simulink model "motorbrushless_simulation"  (R2013a)
settings: Solver=ode4  StartTime=0  StopTime=0.2  FixedStep=Ts  MaxStep=1e-6  RelTol=1e-6  AbsTol=1e-6
PreLoadFcn:
  | assignin('base','Ts',[5e-6])
undefined symbols (not defined in the file or in its folder): Ts
libraries: simulink x19, powerlib_meascontrol x18, powerlib x16
Description:
  | This example illustrates use of the BLDC in a closed-loop
  | speed and voltage control on a 1 kW, 3000 rpm industrial motor
  | 
  | 
  | Copyright 2008-2013 The MathWorks, Inc.
settings Model: ExtModeAutoUpdateStatusClock=off  Creator=MathWorks  LastModifiedBy=Juan Esteban
settings DataIOCC: SignalLoggingSaveFormat=ModelDataLogs  SignalLoggingName=sigsOut
settings OptimizationCC: ExpressionDepthLimit=2147483647  InitFltsAndDblsToZero=on
settings DebuggingCC: SignalResolutionControl=TryResolveAllWithWarning  SolverPrmCheckMsg=none  MultiTaskDSMMsg=warning  MultiTaskCondExecSysMsg=none  FcnCallInpInsideContextMsg=UseLocalSettings
settings HardwareCC: TargetIntDivRoundTo=Zero  TargetEndianess=LittleEndian  TargetHWDeviceType=MATLAB Host  ProdEqTarget=off
settings RTWCC: IncludeERTFirstTime=on
settings GRTTargetCC: CombineOutputUpdateFcns=off  GRTInterface=on

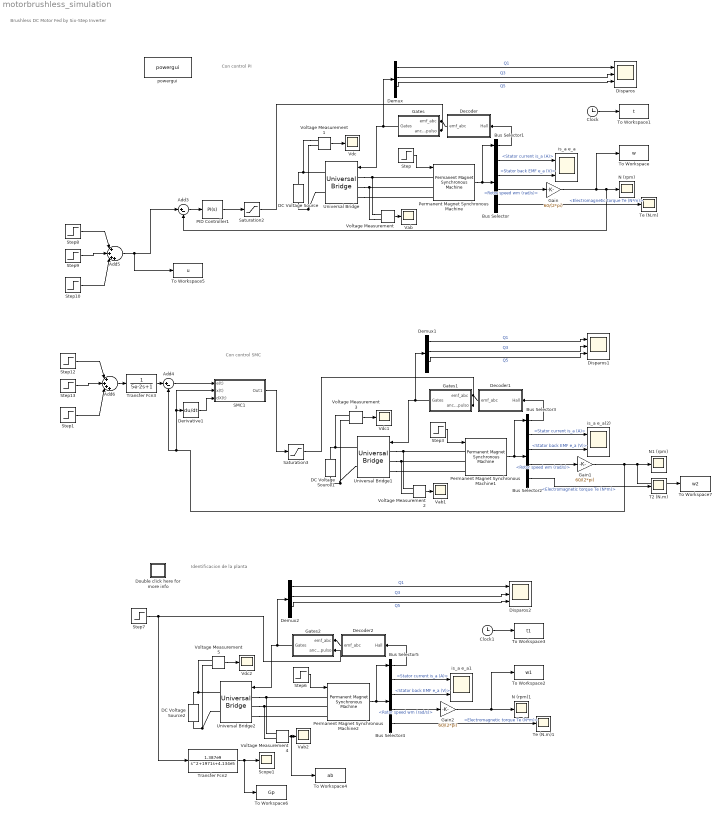
== system motorbrushless_simulation ==
  note: Identificacion de la planta
  note: Con control SMC
  note: Con control PI
  note: Brushless DC Motor Fed by Six-Step Inverter
  Add3 : Sum  Inputs=|+-
  Add4 : Sum  Inputs=|+-
  Add5 : Sum  Inputs=|++++
  Add6 : Sum  Inputs=|++++
  Bus Selector : BusSelector  OutputSignals=Stator current is_a (A),Stator back EMF e_a (V),Rotor speed wm (rad/s),Electromagnetic torque Te (N*m)
  Bus Selector1 : BusSelector  OutputSignals=Hall effect signal h_a,Hall effect signal h_b,Hall effect signal h_c  OutputAsBus=on
  Bus Selector2 : BusSelector  OutputSignals=Stator current is_a (A),Stator back EMF e_a (V),Rotor speed wm (rad/s),Electromagnetic torque Te (N*m)
  Bus Selector3 : BusSelector  OutputSignals=Hall effect signal h_a,Hall effect signal h_b,Hall effect signal h_c  OutputAsBus=on
  Bus Selector4 : BusSelector  OutputSignals=Stator current is_a (A),Stator back EMF e_a (V),Rotor speed wm (rad/s),Electromagnetic torque Te (N*m)
  Bus Selector5 : BusSelector  OutputSignals=Hall effect signal h_a,Hall effect signal h_b,Hall effect signal h_c  OutputAsBus=on
  Clock : Clock
  Clock1 : Clock
  DC Voltage Source : powerlib/Electrical Sources/DC Voltage Source  Amplitude=500  Measurements=None
  DC Voltage Source1 : powerlib/Electrical Sources/DC Voltage Source  Amplitude=500  Measurements=None
  DC Voltage Source2 : powerlib/Electrical Sources/DC Voltage Source  Amplitude=500  Measurements=None
  Decoder : Subsystem
  Decoder1 : Subsystem
  Decoder2 : Subsystem
  Demux : Demux  Outputs=6
  Demux1 : Demux  Outputs=6
  Demux2 : Demux  Outputs=6
  Derivative1 : Derivative
  Disparos : Scope  NumInputPorts=3
      settings: TimeRange=0.2  YMin=0~-5~-5  YMax=500~5~5  DataFormat=Structure
  Disparos1 : Scope  NumInputPorts=3
      settings: TimeRange=0.2  YMin=0~-5~-5  YMax=500~5~5  DataFormat=Structure
  Disparos2 : Scope  NumInputPorts=3
      settings: TimeRange=0.2  YMin=0~-5~-5  YMax=500~5~5  SaveName=ScopeData6  DataFormat=Structure
  Double click here for more info : Subsystem
      settings: OpenFcn=showdemo(bdroot(gcb))
      mask Display: disp('?')
  Gain : Gain  Gain=60/(2*pi)
  Gain1 : Gain  Gain=60/(2*pi)
  Gain2 : Gain  Gain=60/(2*pi)
  Gates : Subsystem
  Gates1 : Subsystem
  Gates2 : Subsystem
  N (rpm) : Scope
      settings: TimeRange=0.2  YMin=0  YMax=3500  SaveName=N
  N (rpm)1 : Scope
      settings: TimeRange=0.2  YMin=2000  YMax=2900  SaveName=N4
  N1 (rpm) : Scope
      settings: TimeRange=0.2  YMin=2040  YMax=2087.5  SaveName=N2
  PID Controller1 : simulink/Continuous/PID Controller  Controller=PI  TimeDomain=Continuous-time  SampleTime=1  IntegratorMethod=Forward Euler  FilterMethod=Forward Euler  Form=Ideal  P=0.000390488448665948  I=609.105574706689  D=0  N=100  InitialConditionSource=internal  InitialConditionForIntegrator=0  InitialConditionForFilter=0  ExternalReset=none  LimitOutput=off  UpperSaturationLimit=inf  LowerSaturationLimit=-inf  LinearizeAsGain=on  AntiWindupMode=none  Kb=1  TrackingMode=off  Kt=1  PParamMin=[]  PParamMax=[]  IParamMin=[]  IParamMax=[]  DParamMin=[]  DParamMax=[]  NParamMin=[]  NParamMax=[]  KbParamMin=[]  KbParamMax=[]  KtParamMin=[]  KtParamMax=[]  POutMin=[]  POutMax=[]  IOutMin=[]  IOutMax=[]  DOutMin=[]  DOutMax=[]  NOutMin=[]  NOutMax=[]  KbOutMin=[]  KbOutMax=[]  KtOutMin=[]  KtOutMax=[]  IntegratorOutMin=[]  IntegratorOutMax=[]  FilterOutMin=[]  FilterOutMax=[]  SumOutMin=[]  SumOutMax=[]  SumI1OutMin=[]  SumI1OutMax=[]  SumI2OutMin=[]  SumI2OutMax=[]  SumI3OutMin=[]  SumI3OutMax=[]  SumDOutMin=[]  SumDOutMax=[]  SaturationOutMin=[]  SaturationOutMax=[]  IntegratorContinuousStateAttributes=''  IntegratorStateMustResolveToSignalObject=off  IntegratorRTWStateStorageClass=Auto  FilterContinuousStateAttributes=''  FilterStateMustResolveToSignalObject=off  FilterRTWStateStorageClass=Auto
  Permanent Magnet Synchronous Machine : powerlib/Machines/Permanent Magnet Synchronous Machine  NbPhases=3  FluxDistribution=Trapezoidal  RotorType=Round  MechanicalLoad=Torque Tm  PresetModel=No  ShowDetailedParameters=on  Resistance=2.8750  Inductance=8.5e-3  dqInductances=[8.5e-3, 8.5e-3]  La=0.000835  MachineConstant=Flux linkage established by magnets (V.s)  Flux=0.175  VoltageCst=146.6077  TorqueCst=1.4  Flat=120  Mechanical=[ 0.8e-3, 1e-3 4]  PolePairs=4  InitialConditions=[0,0, 0,0]  InitialConditions5ph=[0 0 0 0 0 0]  TsPowergui=0  TsBlock=-1  RefAngle=90 degrees behind phase A axis (modified Park)
  Permanent Magnet Synchronous Machine1 : powerlib/Machines/Permanent Magnet Synchronous Machine  NbPhases=3  FluxDistribution=Trapezoidal  RotorType=Round  MechanicalLoad=Torque Tm  PresetModel=No  ShowDetailedParameters=on  Resistance=2.8750  Inductance=8.5e-3  dqInductances=[8.5e-3, 8.5e-3]  La=0.000835  MachineConstant=Flux linkage established by magnets (V.s)  Flux=0.175  VoltageCst=146.6077  TorqueCst=1.4  Flat=120  Mechanical=[ 0.8e-3, 1e-3 4]  PolePairs=4  InitialConditions=[0,0, 0,0]  InitialConditions5ph=[0 0 0 0 0 0]  TsPowergui=0  TsBlock=-1  RefAngle=90 degrees behind phase A axis (modified Park)
  Permanent Magnet Synchronous Machine2 : powerlib/Machines/Permanent Magnet Synchronous Machine  NbPhases=3  FluxDistribution=Trapezoidal  RotorType=Round  MechanicalLoad=Torque Tm  PresetModel=No  ShowDetailedParameters=on  Resistance=2.8750  Inductance=8.5e-3  dqInductances=[8.5e-3, 8.5e-3]  La=0.000835  MachineConstant=Flux linkage established by magnets (V.s)  Flux=0.175  VoltageCst=146.6077  TorqueCst=1.4  Flat=120  Mechanical=[ 0.8e-3, 1e-3 4]  PolePairs=4  InitialConditions=[0,0, 0,0]  InitialConditions5ph=[0 0 0 0 0 0]  TsPowergui=0  TsBlock=-1  RefAngle=90 degrees behind phase A axis (modified Park)
  SMC1 : Subsystem  TreatAsAtomicUnit=on
  Saturation2 : Saturate  UpperLimit=1  LowerLimit=0
  Saturation3 : Saturate  UpperLimit=1  LowerLimit=0
  Scope1 : Scope
      settings: SaveName=ScopeData7
  Step : Step  Time=.1  After=0  SampleTime=0
  Step1 : Step  Time=2.4  After=-2500  SampleTime=0
  Step10 : Step  Time=2.4  After=-2500  SampleTime=0
  Step12 : Step  Time=0  After=1000  SampleTime=0
  Step13 : Step  Time=1.2  After=2000  SampleTime=0
  Step3 : Step  Time=.1  After=0  SampleTime=0
  Step6 : Step  Time=.1  After=0  SampleTime=0
  Step7 : Step  Time=0  SampleTime=0
  Step8 : Step  Time=0  After=1000  SampleTime=0
  Step9 : Step  Time=1.2  After=2000  SampleTime=0
  T2 (N.m) : Scope
      settings: TimeRange=0.2  YMin=0  YMax=3500  SaveName=N3
  Te (N.m) : Scope
      settings: TimeRange=0.2  YMin=0  YMax=3500  SaveName=N1
  Te (N.m)1 : Scope
      settings: TimeRange=0.2  YMin=0  YMax=3500  SaveName=N5
  To Workspace : ToWorkspace  VariableName=w  SampleTime=-1
  To Workspace1 : ToWorkspace  VariableName=t  SampleTime=-1
  To Workspace2 : ToWorkspace  VariableName=w1  SampleTime=-1
  To Workspace3 : ToWorkspace  VariableName=t1  SampleTime=-1
  To Workspace4 : ToWorkspace  VariableName=ab  SampleTime=-1
  To Workspace5 : ToWorkspace  VariableName=u  SampleTime=-1
  To Workspace6 : ToWorkspace  VariableName=Gp  SampleTime=-1
  To Workspace7 : ToWorkspace  VariableName=w2  SampleTime=-1
  Transfer Fcn2 : TransferFcn  Numerator=[1.387e9]  Denominator=[1 1971 4.134e5]
  Transfer Fcn3 : TransferFcn  Denominator=[5e-2 1]
  Universal Bridge : powerlib/Power Electronics/Universal Bridge  Arms=3  SnubberResistance=5000  SnubberCapacitance=1e-6  Device=MOSFET / Diodes  Ron=1e-3  Lon=0  ForwardVoltages="[  0  0  ]"  ForwardVoltage=0  GTOparameters=[ 10e-6 , 20e-6 ]  IGBTparameters=[ 1e-6 , 2e-6 ]  Measurements=None  Measurements_2=None  converterType=Rectifier
  Universal Bridge1 : powerlib/Power Electronics/Universal Bridge  Arms=3  SnubberResistance=5000  SnubberCapacitance=1e-6  Device=MOSFET / Diodes  Ron=1e-3  Lon=0  ForwardVoltages="[  0  0  ]"  ForwardVoltage=0  GTOparameters=[ 10e-6 , 20e-6 ]  IGBTparameters=[ 1e-6 , 2e-6 ]  Measurements=None  Measurements_2=None  converterType=Rectifier
  Universal Bridge2 : powerlib/Power Electronics/Universal Bridge  Arms=3  SnubberResistance=5000  SnubberCapacitance=1e-6  Device=MOSFET / Diodes  Ron=1e-3  Lon=0  ForwardVoltages="[  0  0  ]"  ForwardVoltage=0  GTOparameters=[ 10e-6 , 20e-6 ]  IGBTparameters=[ 1e-6 , 2e-6 ]  Measurements=None  Measurements_2=None  converterType=Rectifier
  Vab : Scope
      settings: TimeRange=0.06  YMin=-10000  YMax=10000  SaveName=ScopeData4  DataFormat=Structure
  Vab1 : Scope
      settings: TimeRange=0.06  YMin=-10000  YMax=10000  SaveName=ScopeData2  DataFormat=Structure
  Vab2 : Scope
      settings: TimeRange=0.06  YMin=-10000  YMax=10000  SaveName=ScopeData8  DataFormat=Structure
  Vdc : Scope
      settings: TimeRange=0.2  YMin=0  YMax=500  SaveName=ScopeData3  DataFormat=Structure
  Vdc1 : Scope
      settings: TimeRange=0.2  YMin=0  YMax=500  SaveName=ScopeData5  DataFormat=Structure
  Vdc2 : Scope
      settings: TimeRange=0.2  YMin=0  YMax=500  SaveName=ScopeData9  DataFormat=Structure
  Voltage Measurement{,1..5} (6 alike) : powerlib/Measurements/Voltage Measurement  PhasorSimulation=off  OutputType=Complex  PSBequivalent=0
  is_a e_a : Scope  NumInputPorts=2
      settings: TimeRange=0.2  YMin=-15~-250  YMax=20~250  SaveName=IE
  is_a e_a(2) : Scope  NumInputPorts=2
      settings: TimeRange=0.2  YMin=-15~-250  YMax=20~250  SaveName=IE1
  is_a e_a1 : Scope  NumInputPorts=2
      settings: TimeRange=0.2  YMin=-15~-250  YMax=20~250  SaveName=IE2
  powergui : powerlib/powergui  Priority=2  SimulationMode=Discrete  SolverType=Tustin  SampleTime=Ts  frequency=60  SPID=off  DisableSnubberDevices=off  DisableRonSwitches=off  DisableVfSwitches=off  SwTol=0  Interpol=off  DisplayEquations=off  frequencyindice=0  Pbase=100e6  ErrMax=1e-4  Iterations=50  UnitsV=kV  UnitsW=MW  FunctionMessages=off  echomessages=off  HookPort=off  EnableUseOfTLC=off  x0status=blocks  RestoreLinks=warning  ResistiveCurrentMeasurement=off  Frange=[0:2:500]  Ylog=off  Xlog=on  ShowGrid=off  save=off  variable=ZData  ZoomFFT=on  StartTime=0.0  cycles=1  DisplayStyle=1  fundamental=60  FreqAxis=off  MaxFrequency=1000  frequencyindicesteady=1  RmsSteady=1  display=off  Ts=0  methode=off
  wires:
  Step/1 -> Permanent Magnet Synchronous Machine/1
  Gates/1(Gates) -> Demux/1, Universal Bridge/1
  Decoder/1(emf_abc) -> Gates/1("emf_abc ")
  Voltage Measurement/1 -> Vab/1
  Voltage Measurement1/1 -> Vdc/1
  Bus Selector/1 -> is_a e_a/1  "<Stator current is_a (A)>"
  Permanent Magnet Synchronous Machine/1 -> Bus Selector/1, Bus Selector1/1
  Bus Selector1/1 -> Decoder/1("Hall ")
  Bus Selector/2 -> is_a e_a/2  "<Stator back EMF e_a (V)>"
  Bus Selector/4 -> Te (N.m)/1  "<Electromagnetic torque Te (N*m)>"
  Bus Selector/3 -> Gain/1  "<Rotor speed wm (rad/s)>"
  Gain/1 -> To Workspace/1, Add3/2, N (rpm)/1
  Clock/1 -> To Workspace1/1
  Add3/1 -> PID Controller1/1
  Demux/1 -> Disparos/1  "Q1"
  Demux/3 -> Disparos/2  "Q3"
  Demux/5 -> Disparos/3  "Q5"
  PID Controller1/1 -> Saturation2/1
  Saturation2/1 -> Gates/2(ancho_pulso)
  Add5/1 -> To Workspace5/1, Add3/1
  Step8/1 -> Add5/1
  Step9/1 -> Add5/2
  Step10/1 -> Add5/3
  Step3/1 -> Permanent Magnet Synchronous Machine1/1
  Gates1/1(Gates) -> Demux1/1, Universal Bridge1/1
  Decoder1/1(emf_abc) -> Gates1/1("emf_abc ")
  Voltage Measurement2/1 -> Vab1/1
  Voltage Measurement3/1 -> Vdc1/1
  Bus Selector2/1 -> is_a e_a(2)/1  "<Stator current is_a (A)>"
  Permanent Magnet Synchronous Machine1/1 -> Bus Selector2/1, Bus Selector3/1
  Bus Selector3/1 -> Decoder1/1("Hall ")
  Bus Selector2/2 -> is_a e_a(2)/2  "<Stator back EMF e_a (V)>"
  Bus Selector2/4 -> T2 (N.m)/1  "<Electromagnetic torque Te (N*m)>"
  Bus Selector2/3 -> Gain1/1  "<Rotor speed wm (rad/s)>"
  Demux1/1 -> Disparos1/1  "Q1"
  Demux1/3 -> Disparos1/2  "Q3"
  Demux1/5 -> Disparos1/3  "Q5"
  Add4/1 -> SMC1/1(e(t))
  Derivative1/1 -> SMC1/3(dX(t))
  Gain1/1 -> Derivative1/1, SMC1/2(x(t)), Add4/2, To Workspace7/1, N1 (rpm)/1
  SMC1/1(Out1) -> Saturation3/1
  Saturation3/1 -> Gates1/2(ancho_pulso)
  Step12/1 -> Add6/1
  Step13/1 -> Add6/2
  Step1/1 -> Add6/3
  Transfer Fcn3/1 -> Add4/1
  Add6/1 -> Transfer Fcn3/1
  Step6/1 -> Permanent Magnet Synchronous Machine2/1
  Gates2/1(Gates) -> Demux2/1, Universal Bridge2/1
  Decoder2/1(emf_abc) -> Gates2/1("emf_abc ")
  Voltage Measurement4/1 -> To Workspace4/1, Vab2/1
  Voltage Measurement5/1 -> Vdc2/1
  Bus Selector4/1 -> is_a e_a1/1  "<Stator current is_a (A)>"
  Permanent Magnet Synchronous Machine2/1 -> Bus Selector4/1, Bus Selector5/1
  Bus Selector5/1 -> Decoder2/1("Hall ")
  Bus Selector4/2 -> is_a e_a1/2  "<Stator back EMF e_a (V)>"
  Bus Selector4/4 -> Te (N.m)1/1  "<Electromagnetic torque Te (N*m)>"
  Bus Selector4/3 -> Gain2/1  "<Rotor speed wm (rad/s)>"
  Gain2/1 -> To Workspace2/1, N (rpm)1/1
  Clock1/1 -> To Workspace3/1
  Demux2/1 -> Disparos2/1  "Q1"
  Demux2/3 -> Disparos2/2  "Q3"
  Demux2/5 -> Disparos2/3  "Q5"
  Step7/1 -> Transfer Fcn2/1, Gates2/2(ancho_pulso)
  Transfer Fcn2/1 -> To Workspace6/1, Scope1/1
  connections:
  Voltage Measurement/LConn1 -- Permanent Magnet Synchronous Machine/LConn1 -- Universal Bridge/LConn1
  Voltage Measurement/LConn2 -- Permanent Magnet Synchronous Machine/LConn2 -- Universal Bridge/LConn2
  Voltage Measurement1/LConn1 -- Universal Bridge/RConn1 -- DC Voltage Source/RConn1
  Voltage Measurement1/LConn2 -- Universal Bridge/RConn2 -- DC Voltage Source/LConn1
  Universal Bridge/LConn3 -- Permanent Magnet Synchronous Machine/LConn3
  Universal Bridge1/LConn1 -- Voltage Measurement2/LConn1 -- Permanent Magnet Synchronous Machine1/LConn1
  Universal Bridge1/LConn2 -- Voltage Measurement2/LConn2 -- Permanent Magnet Synchronous Machine1/LConn2
  DC Voltage Source1/RConn1 -- Voltage Measurement3/LConn1 -- Universal Bridge1/RConn1
  DC Voltage Source1/LConn1 -- Voltage Measurement3/LConn2 -- Universal Bridge1/RConn2
  Universal Bridge1/LConn3 -- Permanent Magnet Synchronous Machine1/LConn3
  Universal Bridge2/LConn1 -- Voltage Measurement4/LConn1 -- Permanent Magnet Synchronous Machine2/LConn1
  Universal Bridge2/LConn2 -- Voltage Measurement4/LConn2 -- Permanent Magnet Synchronous Machine2/LConn2
  DC Voltage Source2/RConn1 -- Voltage Measurement5/LConn1 -- Universal Bridge2/RConn1
  DC Voltage Source2/LConn1 -- Voltage Measurement5/LConn2 -- Universal Bridge2/RConn2
  Universal Bridge2/LConn3 -- Permanent Magnet Synchronous Machine2/LConn3

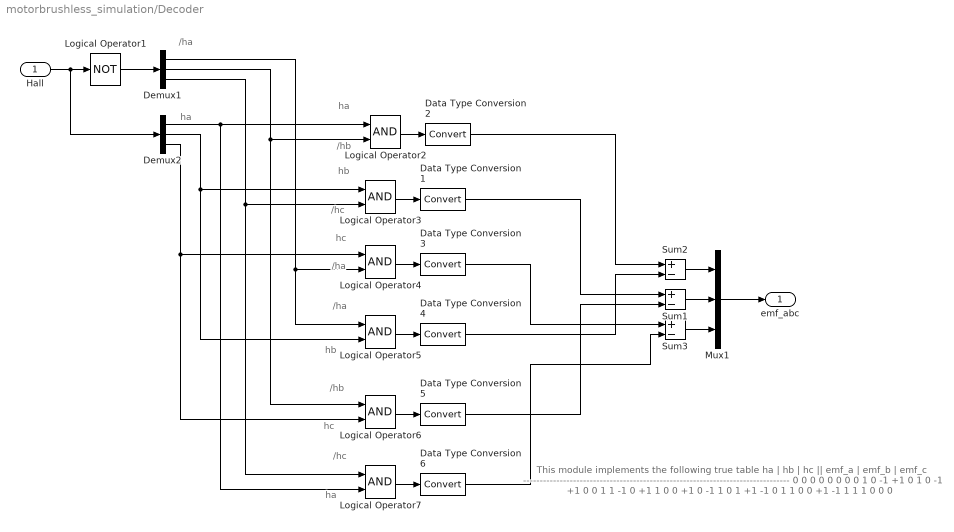
== system motorbrushless_simulation/Decoder ==
  note: /ha
  note: ha
  note: ha
  note: /hb
  note: hb
  note: /hc
  note: hc
  note: /ha
  note: /ha
  note: hb
  note: /hb
  note: hc
  note: /hc
  note: ha
  note: This module implements the following true table
      |
      |    ha   |   hb   |   hc   ||   emf_a   |   emf_b   |   emf_c
      |     --------------------------------------------------------------------------------
      | 0          0         0          0               0               0
      | 0          0         1          0               -1              +1
      | 0          1         0          -1              +1                0
      | 0          1         1          -1               0               +1
      | 1          0         0         +1               0               -1
      | 1          0         1         +1              -1                0
      | 1          1         0          0              +1               -1
      | 1          1         1          0               0                0
  "Hall " : Inport
  Data Type Conversion{1..6} (6 alike) : DataTypeConversion
  Demux1 : Demux  Outputs=3
  Demux2 : Demux  Outputs=3
  Logical Operator1 : Logic  Operator=NOT  AllPortsSameDT=off  OutDataTypeStr=boolean
  Logical Operator{2..7} (6 alike) : Logic  AllPortsSameDT=off  OutDataTypeStr=boolean
  Mux1 : Mux  Inputs=3
  Sum1 : Sum  Inputs=+-  OutDataTypeStr=double
  Sum2 : Sum  Inputs=+-  OutDataTypeStr=double
  Sum3 : Sum  Inputs=+-  OutDataTypeStr=double
  emf_abc : Outport
  wires:
  "Hall "/1 -> Logical Operator1/1, Demux2/1
  Logical Operator1/1 -> Demux1/1
  Demux2/3 -> Logical Operator4/1, Logical Operator6/2
  Demux2/2 -> Logical Operator3/1, Logical Operator5/2
  Demux2/1 -> Logical Operator2/1, Logical Operator7/2
  Demux1/3 -> Logical Operator3/2, Logical Operator7/1
  Demux1/2 -> Logical Operator2/2, Logical Operator6/1
  Demux1/1 -> Logical Operator4/2, Logical Operator5/1
  Logical Operator2/1 -> Data Type Conversion2/1
  Sum2/1 -> Mux1/1
  Sum1/1 -> Mux1/2
  Sum3/1 -> Mux1/3
  Mux1/1 -> emf_abc/1
  Logical Operator3/1 -> Data Type Conversion1/1
  Logical Operator4/1 -> Data Type Conversion3/1
  Logical Operator5/1 -> Data Type Conversion4/1
  Logical Operator6/1 -> Data Type Conversion5/1
  Logical Operator7/1 -> Data Type Conversion6/1
  Data Type Conversion2/1 -> Sum2/1
  Data Type Conversion4/1 -> Sum2/2
  Data Type Conversion1/1 -> Sum1/1
  Data Type Conversion5/1 -> Sum1/2
  Data Type Conversion3/1 -> Sum3/1
  Data Type Conversion6/1 -> Sum3/2

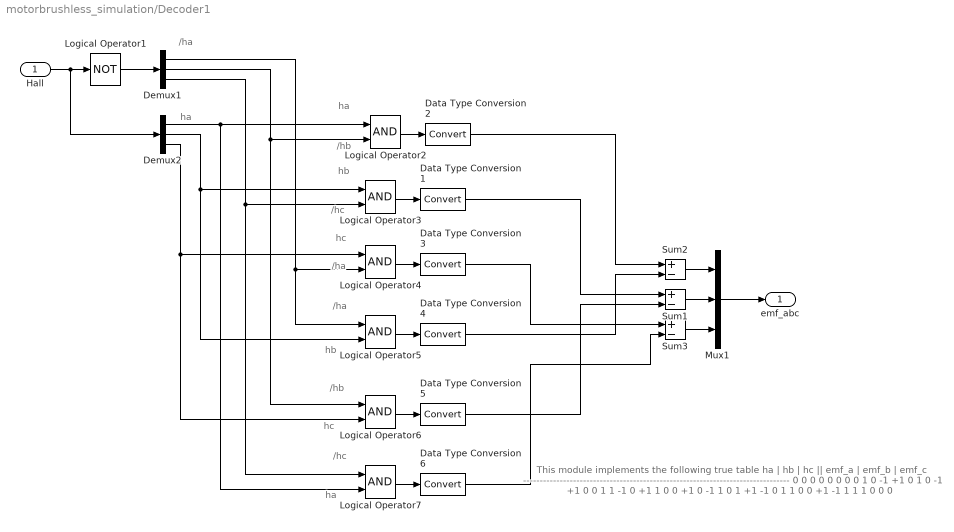
== system motorbrushless_simulation/Decoder1 ==
  note: /ha
  note: ha
  note: ha
  note: /hb
  note: hb
  note: /hc
  note: hc
  note: /ha
  note: /ha
  note: hb
  note: /hb
  note: hc
  note: /hc
  note: ha
  note: This module implements the following true table
      |
      |    ha   |   hb   |   hc   ||   emf_a   |   emf_b   |   emf_c
      |     --------------------------------------------------------------------------------
      | 0          0         0          0               0               0
      | 0          0         1          0               -1              +1
      | 0          1         0          -1              +1                0
      | 0          1         1          -1               0               +1
      | 1          0         0         +1               0               -1
      | 1          0         1         +1              -1                0
      | 1          1         0          0              +1               -1
      | 1          1         1          0               0                0
  "Hall " : Inport
  Data Type Conversion{1..6} (6 alike) : DataTypeConversion
  Demux1 : Demux  Outputs=3
  Demux2 : Demux  Outputs=3
  Logical Operator1 : Logic  Operator=NOT  AllPortsSameDT=off  OutDataTypeStr=boolean
  Logical Operator{2..7} (6 alike) : Logic  AllPortsSameDT=off  OutDataTypeStr=boolean
  Mux1 : Mux  Inputs=3
  Sum1 : Sum  Inputs=+-  OutDataTypeStr=double
  Sum2 : Sum  Inputs=+-  OutDataTypeStr=double
  Sum3 : Sum  Inputs=+-  OutDataTypeStr=double
  emf_abc : Outport
  wires:
  "Hall "/1 -> Logical Operator1/1, Demux2/1
  Logical Operator1/1 -> Demux1/1
  Demux2/3 -> Logical Operator4/1, Logical Operator6/2
  Demux2/2 -> Logical Operator3/1, Logical Operator5/2
  Demux2/1 -> Logical Operator2/1, Logical Operator7/2
  Demux1/3 -> Logical Operator3/2, Logical Operator7/1
  Demux1/2 -> Logical Operator2/2, Logical Operator6/1
  Demux1/1 -> Logical Operator4/2, Logical Operator5/1
  Logical Operator2/1 -> Data Type Conversion2/1
  Sum2/1 -> Mux1/1
  Sum1/1 -> Mux1/2
  Sum3/1 -> Mux1/3
  Mux1/1 -> emf_abc/1
  Logical Operator3/1 -> Data Type Conversion1/1
  Logical Operator4/1 -> Data Type Conversion3/1
  Logical Operator5/1 -> Data Type Conversion4/1
  Logical Operator6/1 -> Data Type Conversion5/1
  Logical Operator7/1 -> Data Type Conversion6/1
  Data Type Conversion2/1 -> Sum2/1
  Data Type Conversion4/1 -> Sum2/2
  Data Type Conversion1/1 -> Sum1/1
  Data Type Conversion5/1 -> Sum1/2
  Data Type Conversion3/1 -> Sum3/1
  Data Type Conversion6/1 -> Sum3/2

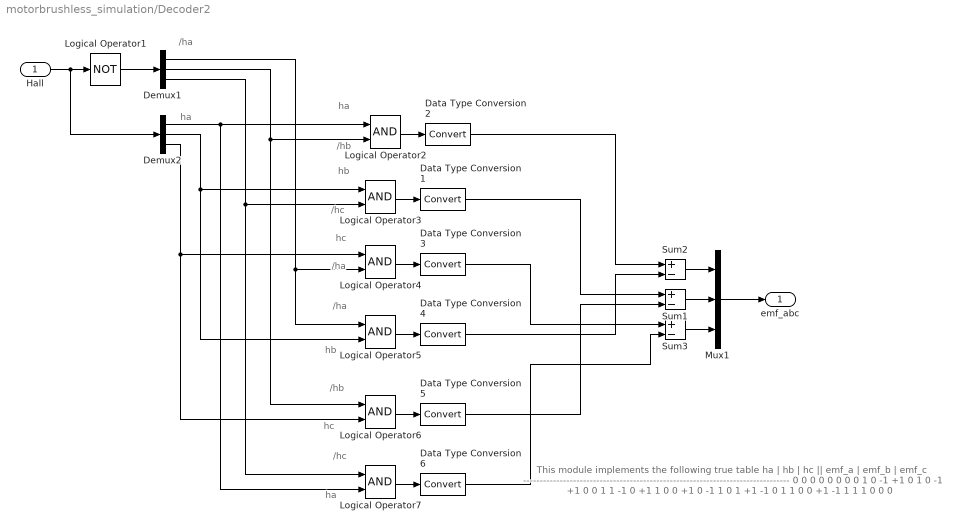
== system motorbrushless_simulation/Decoder2 ==
  note: /ha
  note: ha
  note: ha
  note: /hb
  note: hb
  note: /hc
  note: hc
  note: /ha
  note: /ha
  note: hb
  note: /hb
  note: hc
  note: /hc
  note: ha
  note: This module implements the following true table
      |
      |    ha   |   hb   |   hc   ||   emf_a   |   emf_b   |   emf_c
      |     --------------------------------------------------------------------------------
      | 0          0         0          0               0               0
      | 0          0         1          0               -1              +1
      | 0          1         0          -1              +1                0
      | 0          1         1          -1               0               +1
      | 1          0         0         +1               0               -1
      | 1          0         1         +1              -1                0
      | 1          1         0          0              +1               -1
      | 1          1         1          0               0                0
  "Hall " : Inport
  Data Type Conversion{1..6} (6 alike) : DataTypeConversion
  Demux1 : Demux  Outputs=3
  Demux2 : Demux  Outputs=3
  Logical Operator1 : Logic  Operator=NOT  AllPortsSameDT=off  OutDataTypeStr=boolean
  Logical Operator{2..7} (6 alike) : Logic  AllPortsSameDT=off  OutDataTypeStr=boolean
  Mux1 : Mux  Inputs=3
  Sum1 : Sum  Inputs=+-  OutDataTypeStr=double
  Sum2 : Sum  Inputs=+-  OutDataTypeStr=double
  Sum3 : Sum  Inputs=+-  OutDataTypeStr=double
  emf_abc : Outport
  wires:
  "Hall "/1 -> Logical Operator1/1, Demux2/1
  Logical Operator1/1 -> Demux1/1
  Demux2/3 -> Logical Operator4/1, Logical Operator6/2
  Demux2/2 -> Logical Operator3/1, Logical Operator5/2
  Demux2/1 -> Logical Operator2/1, Logical Operator7/2
  Demux1/3 -> Logical Operator3/2, Logical Operator7/1
  Demux1/2 -> Logical Operator2/2, Logical Operator6/1
  Demux1/1 -> Logical Operator4/2, Logical Operator5/1
  Logical Operator2/1 -> Data Type Conversion2/1
  Sum2/1 -> Mux1/1
  Sum1/1 -> Mux1/2
  Sum3/1 -> Mux1/3
  Mux1/1 -> emf_abc/1
  Logical Operator3/1 -> Data Type Conversion1/1
  Logical Operator4/1 -> Data Type Conversion3/1
  Logical Operator5/1 -> Data Type Conversion4/1
  Logical Operator6/1 -> Data Type Conversion5/1
  Logical Operator7/1 -> Data Type Conversion6/1
  Data Type Conversion2/1 -> Sum2/1
  Data Type Conversion4/1 -> Sum2/2
  Data Type Conversion1/1 -> Sum1/1
  Data Type Conversion5/1 -> Sum1/2
  Data Type Conversion3/1 -> Sum3/1
  Data Type Conversion6/1 -> Sum3/2

== system motorbrushless_simulation/Double click here for more info ==

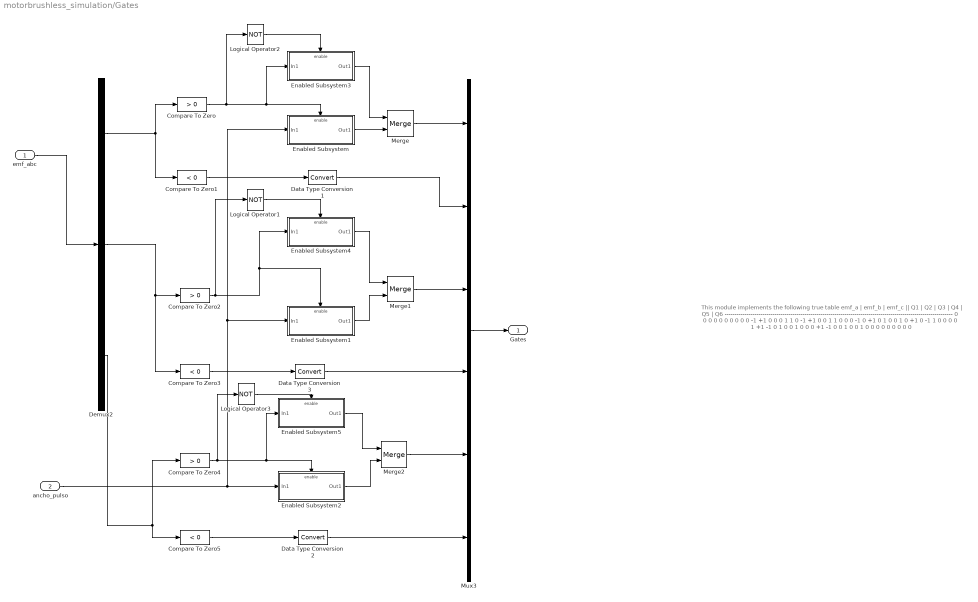
== system motorbrushless_simulation/Gates ==
  note: This module implements the following true table
      |
      |    emf_a   |   emf_b   |   emf_c   ||   Q1   |   Q2   |   Q3   |   Q4   |   Q5   |   Q6
      |     ------------------------------------------------------------------------------------------------------------------
      |       0              0                0            0          0          0           0        0        0
      |       0               -1              +1          0          0          0           1        1        0
      |     -1              +1                0          0          1          1           0        0        0
      |     -1               0               +1          0          1         0           0        1        0
      |    +1               0                -1          1          0          0           0        0        1
      |    +1              -1                0           1          0          0           1        0        0
      |      0              +1               -1           0          0          1           0        0        1
      |     0              0                0             0          0          0           0        0        0
  "emf_abc " : Inport
  ancho_pulso : Inport  Port=2
  Compare To Zero : simulink/Logic and Bit Operations/Compare To Zero  relop=>  OutDataTypeStr=boolean  ZeroCross=off
  Compare To Zero1 : simulink/Logic and Bit Operations/Compare To Zero  relop=<  OutDataTypeStr=boolean  ZeroCross=off
  Compare To Zero2 : simulink/Logic and Bit Operations/Compare To Zero  relop=>  OutDataTypeStr=boolean  ZeroCross=off
  Compare To Zero3 : simulink/Logic and Bit Operations/Compare To Zero  relop=<  OutDataTypeStr=boolean  ZeroCross=off
  Compare To Zero4 : simulink/Logic and Bit Operations/Compare To Zero  relop=>  OutDataTypeStr=boolean  ZeroCross=off
  Compare To Zero5 : simulink/Logic and Bit Operations/Compare To Zero  relop=<  OutDataTypeStr=boolean  ZeroCross=off
  Data Type Conversion1 : DataTypeConversion
  Data Type Conversion2 : DataTypeConversion
  Data Type Conversion3 : DataTypeConversion
  Demux2 : Demux  Outputs=3
  Enabled Subsystem : Subsystem  TreatAsAtomicUnit=on
  Enabled Subsystem1 : Subsystem  TreatAsAtomicUnit=on
  Enabled Subsystem2 : Subsystem  TreatAsAtomicUnit=on
  Enabled Subsystem3 : Subsystem  TreatAsAtomicUnit=on
  Enabled Subsystem4 : Subsystem  TreatAsAtomicUnit=on
  Enabled Subsystem5 : Subsystem  TreatAsAtomicUnit=on
  Logical Operator1 : Logic  Operator=NOT  Inputs=3  AllPortsSameDT=off  OutDataTypeStr=boolean
  Logical Operator2 : Logic  Operator=NOT  Inputs=3  AllPortsSameDT=off  OutDataTypeStr=boolean
  Logical Operator3 : Logic  Operator=NOT  Inputs=3  AllPortsSameDT=off  OutDataTypeStr=boolean
  Merge : Merge
  Merge1 : Merge
  Merge2 : Merge
  Mux3 : Mux  Inputs=6
  Gates : Outport
  wires:
  "emf_abc "/1 -> Demux2/1
  Mux3/1 -> Gates/1
  Demux2/1 -> Compare To Zero/1, Compare To Zero1/1
  Demux2/2 -> Compare To Zero2/1, Compare To Zero3/1
  Demux2/3 -> Compare To Zero4/1, Compare To Zero5/1
  Compare To Zero/1 -> Logical Operator2/1, Enabled Subsystem3/1(In1), Enabled Subsystem/Enable
  Enabled Subsystem/1(Out1) -> Merge/2
  Merge/1 -> Mux3/1
  Enabled Subsystem1/1(Out1) -> Merge1/2
  Merge1/1 -> Mux3/3
  Enabled Subsystem2/1(Out1) -> Merge2/2
  Merge2/1 -> Mux3/5
  Logical Operator2/1 -> Enabled Subsystem3/Enable
  Enabled Subsystem3/1(Out1) -> Merge/1
  Compare To Zero1/1 -> Data Type Conversion1/1
  Data Type Conversion1/1 -> Mux3/2
  Compare To Zero2/1 -> Enabled Subsystem4/1(In1), Enabled Subsystem1/Enable, Logical Operator1/1
  Logical Operator1/1 -> Enabled Subsystem4/Enable
  Enabled Subsystem4/1(Out1) -> Merge1/1
  Data Type Conversion3/1 -> Mux3/4
  Compare To Zero3/1 -> Data Type Conversion3/1
  Compare To Zero4/1 -> Logical Operator3/1, Enabled Subsystem5/1(In1), Enabled Subsystem2/Enable
  Logical Operator3/1 -> Enabled Subsystem5/Enable
  Compare To Zero5/1 -> Data Type Conversion2/1
  Data Type Conversion2/1 -> Mux3/6
  ancho_pulso/1 -> Enabled Subsystem1/1(In1), Enabled Subsystem/1(In1), Enabled Subsystem2/1(In1)
  Enabled Subsystem5/1(Out1) -> Merge2/1

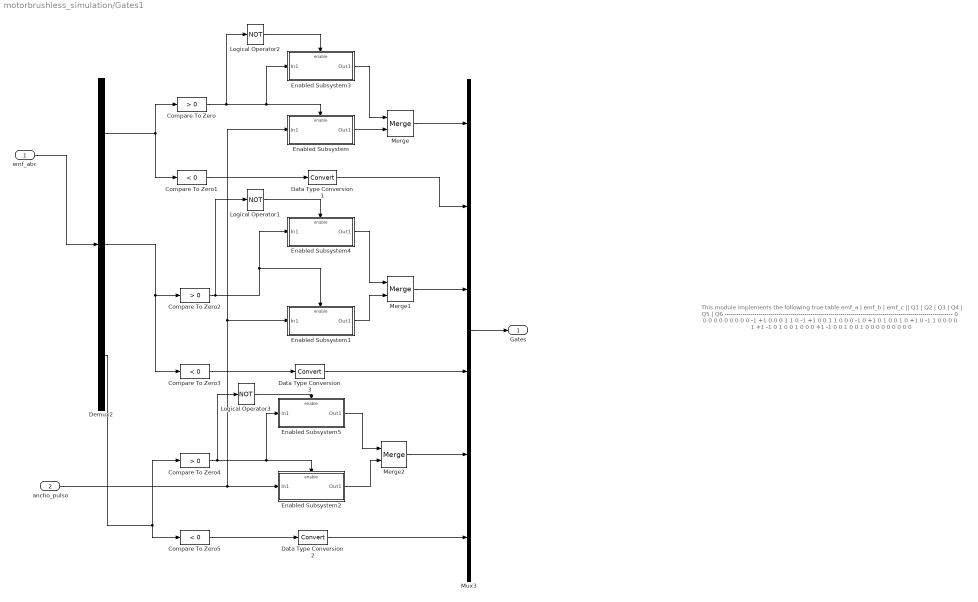
== system motorbrushless_simulation/Gates1 ==
  note: This module implements the following true table
      |
      |    emf_a   |   emf_b   |   emf_c   ||   Q1   |   Q2   |   Q3   |   Q4   |   Q5   |   Q6
      |     ------------------------------------------------------------------------------------------------------------------
      |       0              0                0            0          0          0           0        0        0
      |       0               -1              +1          0          0          0           1        1        0
      |     -1              +1                0          0          1          1           0        0        0
      |     -1               0               +1          0          1         0           0        1        0
      |    +1               0                -1          1          0          0           0        0        1
      |    +1              -1                0           1          0          0           1        0        0
      |      0              +1               -1           0          0          1           0        0        1
      |     0              0                0             0          0          0           0        0        0
  "emf_abc " : Inport
  ancho_pulso : Inport  Port=2
  Compare To Zero : simulink/Logic and Bit Operations/Compare To Zero  relop=>  OutDataTypeStr=boolean  ZeroCross=off
  Compare To Zero1 : simulink/Logic and Bit Operations/Compare To Zero  relop=<  OutDataTypeStr=boolean  ZeroCross=off
  Compare To Zero2 : simulink/Logic and Bit Operations/Compare To Zero  relop=>  OutDataTypeStr=boolean  ZeroCross=off
  Compare To Zero3 : simulink/Logic and Bit Operations/Compare To Zero  relop=<  OutDataTypeStr=boolean  ZeroCross=off
  Compare To Zero4 : simulink/Logic and Bit Operations/Compare To Zero  relop=>  OutDataTypeStr=boolean  ZeroCross=off
  Compare To Zero5 : simulink/Logic and Bit Operations/Compare To Zero  relop=<  OutDataTypeStr=boolean  ZeroCross=off
  Data Type Conversion1 : DataTypeConversion
  Data Type Conversion2 : DataTypeConversion
  Data Type Conversion3 : DataTypeConversion
  Demux2 : Demux  Outputs=3
  Enabled Subsystem : Subsystem  TreatAsAtomicUnit=on
  Enabled Subsystem1 : Subsystem  TreatAsAtomicUnit=on
  Enabled Subsystem2 : Subsystem  TreatAsAtomicUnit=on
  Enabled Subsystem3 : Subsystem  TreatAsAtomicUnit=on
  Enabled Subsystem4 : Subsystem  TreatAsAtomicUnit=on
  Enabled Subsystem5 : Subsystem  TreatAsAtomicUnit=on
  Logical Operator1 : Logic  Operator=NOT  Inputs=3  AllPortsSameDT=off  OutDataTypeStr=boolean
  Logical Operator2 : Logic  Operator=NOT  Inputs=3  AllPortsSameDT=off  OutDataTypeStr=boolean
  Logical Operator3 : Logic  Operator=NOT  Inputs=3  AllPortsSameDT=off  OutDataTypeStr=boolean
  Merge : Merge
  Merge1 : Merge
  Merge2 : Merge
  Mux3 : Mux  Inputs=6
  Gates : Outport
  wires:
  "emf_abc "/1 -> Demux2/1
  Mux3/1 -> Gates/1
  Demux2/1 -> Compare To Zero/1, Compare To Zero1/1
  Demux2/2 -> Compare To Zero2/1, Compare To Zero3/1
  Demux2/3 -> Compare To Zero4/1, Compare To Zero5/1
  Compare To Zero/1 -> Logical Operator2/1, Enabled Subsystem3/1(In1), Enabled Subsystem/Enable
  Enabled Subsystem/1(Out1) -> Merge/2
  Merge/1 -> Mux3/1
  Enabled Subsystem1/1(Out1) -> Merge1/2
  Merge1/1 -> Mux3/3
  Enabled Subsystem2/1(Out1) -> Merge2/2
  Merge2/1 -> Mux3/5
  Logical Operator2/1 -> Enabled Subsystem3/Enable
  Enabled Subsystem3/1(Out1) -> Merge/1
  Compare To Zero1/1 -> Data Type Conversion1/1
  Data Type Conversion1/1 -> Mux3/2
  Compare To Zero2/1 -> Enabled Subsystem4/1(In1), Enabled Subsystem1/Enable, Logical Operator1/1
  Logical Operator1/1 -> Enabled Subsystem4/Enable
  Enabled Subsystem4/1(Out1) -> Merge1/1
  Data Type Conversion3/1 -> Mux3/4
  Compare To Zero3/1 -> Data Type Conversion3/1
  Compare To Zero4/1 -> Logical Operator3/1, Enabled Subsystem5/1(In1), Enabled Subsystem2/Enable
  Logical Operator3/1 -> Enabled Subsystem5/Enable
  Compare To Zero5/1 -> Data Type Conversion2/1
  Data Type Conversion2/1 -> Mux3/6
  ancho_pulso/1 -> Enabled Subsystem1/1(In1), Enabled Subsystem/1(In1), Enabled Subsystem2/1(In1)
  Enabled Subsystem5/1(Out1) -> Merge2/1

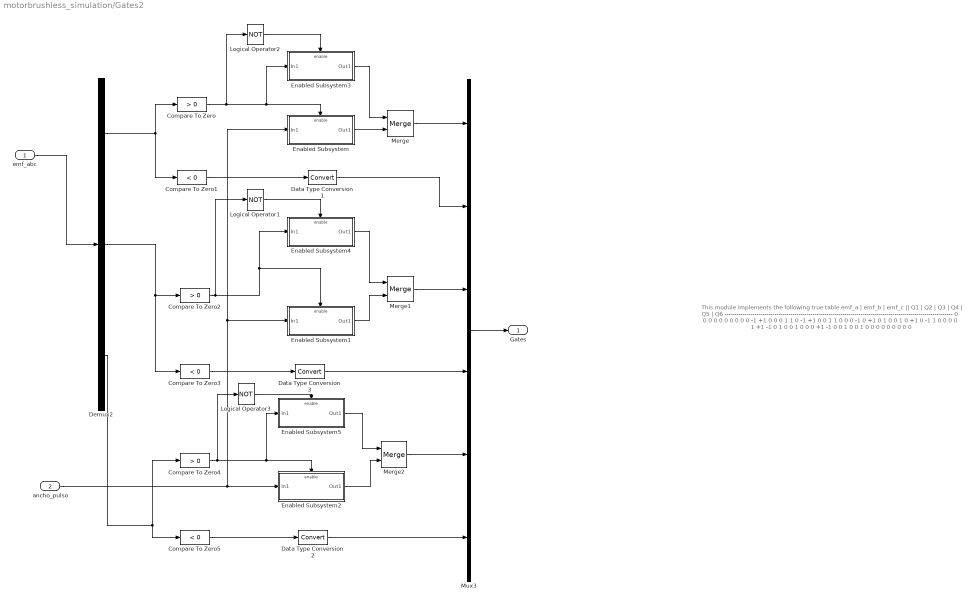
== system motorbrushless_simulation/Gates2 ==
  note: This module implements the following true table
      |
      |    emf_a   |   emf_b   |   emf_c   ||   Q1   |   Q2   |   Q3   |   Q4   |   Q5   |   Q6
      |     ------------------------------------------------------------------------------------------------------------------
      |       0              0                0            0          0          0           0        0        0
      |       0               -1              +1          0          0          0           1        1        0
      |     -1              +1                0          0          1          1           0        0        0
      |     -1               0               +1          0          1         0           0        1        0
      |    +1               0                -1          1          0          0           0        0        1
      |    +1              -1                0           1          0          0           1        0        0
      |      0              +1               -1           0          0          1           0        0        1
      |     0              0                0             0          0          0           0        0        0
  "emf_abc " : Inport
  ancho_pulso : Inport  Port=2
  Compare To Zero : simulink/Logic and Bit Operations/Compare To Zero  relop=>  OutDataTypeStr=boolean  ZeroCross=off
  Compare To Zero1 : simulink/Logic and Bit Operations/Compare To Zero  relop=<  OutDataTypeStr=boolean  ZeroCross=off
  Compare To Zero2 : simulink/Logic and Bit Operations/Compare To Zero  relop=>  OutDataTypeStr=boolean  ZeroCross=off
  Compare To Zero3 : simulink/Logic and Bit Operations/Compare To Zero  relop=<  OutDataTypeStr=boolean  ZeroCross=off
  Compare To Zero4 : simulink/Logic and Bit Operations/Compare To Zero  relop=>  OutDataTypeStr=boolean  ZeroCross=off
  Compare To Zero5 : simulink/Logic and Bit Operations/Compare To Zero  relop=<  OutDataTypeStr=boolean  ZeroCross=off
  Data Type Conversion1 : DataTypeConversion
  Data Type Conversion2 : DataTypeConversion
  Data Type Conversion3 : DataTypeConversion
  Demux2 : Demux  Outputs=3
  Enabled Subsystem : Subsystem  TreatAsAtomicUnit=on
  Enabled Subsystem1 : Subsystem  TreatAsAtomicUnit=on
  Enabled Subsystem2 : Subsystem  TreatAsAtomicUnit=on
  Enabled Subsystem3 : Subsystem  TreatAsAtomicUnit=on
  Enabled Subsystem4 : Subsystem  TreatAsAtomicUnit=on
  Enabled Subsystem5 : Subsystem  TreatAsAtomicUnit=on
  Logical Operator1 : Logic  Operator=NOT  Inputs=3  AllPortsSameDT=off  OutDataTypeStr=boolean
  Logical Operator2 : Logic  Operator=NOT  Inputs=3  AllPortsSameDT=off  OutDataTypeStr=boolean
  Logical Operator3 : Logic  Operator=NOT  Inputs=3  AllPortsSameDT=off  OutDataTypeStr=boolean
  Merge : Merge
  Merge1 : Merge
  Merge2 : Merge
  Mux3 : Mux  Inputs=6
  Gates : Outport
  wires:
  "emf_abc "/1 -> Demux2/1
  Mux3/1 -> Gates/1
  Demux2/1 -> Compare To Zero/1, Compare To Zero1/1
  Demux2/2 -> Compare To Zero2/1, Compare To Zero3/1
  Demux2/3 -> Compare To Zero4/1, Compare To Zero5/1
  Compare To Zero/1 -> Logical Operator2/1, Enabled Subsystem3/1(In1), Enabled Subsystem/Enable
  Enabled Subsystem/1(Out1) -> Merge/2
  Merge/1 -> Mux3/1
  Enabled Subsystem1/1(Out1) -> Merge1/2
  Merge1/1 -> Mux3/3
  Enabled Subsystem2/1(Out1) -> Merge2/2
  Merge2/1 -> Mux3/5
  Logical Operator2/1 -> Enabled Subsystem3/Enable
  Enabled Subsystem3/1(Out1) -> Merge/1
  Compare To Zero1/1 -> Data Type Conversion1/1
  Data Type Conversion1/1 -> Mux3/2
  Compare To Zero2/1 -> Enabled Subsystem4/1(In1), Enabled Subsystem1/Enable, Logical Operator1/1
  Logical Operator1/1 -> Enabled Subsystem4/Enable
  Enabled Subsystem4/1(Out1) -> Merge1/1
  Data Type Conversion3/1 -> Mux3/4
  Compare To Zero3/1 -> Data Type Conversion3/1
  Compare To Zero4/1 -> Logical Operator3/1, Enabled Subsystem5/1(In1), Enabled Subsystem2/Enable
  Logical Operator3/1 -> Enabled Subsystem5/Enable
  Compare To Zero5/1 -> Data Type Conversion2/1
  Data Type Conversion2/1 -> Mux3/6
  ancho_pulso/1 -> Enabled Subsystem1/1(In1), Enabled Subsystem/1(In1), Enabled Subsystem2/1(In1)
  Enabled Subsystem5/1(Out1) -> Merge2/1

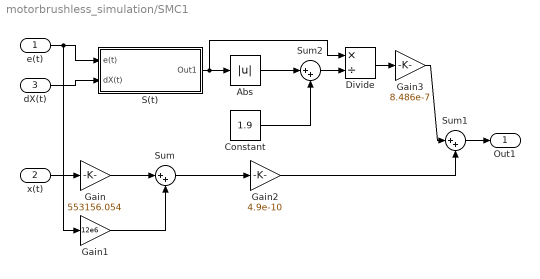
== system motorbrushless_simulation/SMC1 ==
  e(t) : Inport
  x(t) : Inport  Port=2
  dX(t) : Inport  Port=3
  Abs : Abs
  Constant : Constant  Value=1.9
  Divide : Product  Inputs=*/
  Gain : Gain  Gain=553156.054
  Gain1 : Gain  Gain=12e6
  Gain2 : Gain  Gain=4.9e-10
  Gain3 : Gain  Gain=8.486e-7
  S(t) : Subsystem  TreatAsAtomicUnit=on
  Sum : Sum  Inputs=|++
  Sum1 : Sum  Inputs=|++
  Sum2 : Sum  Inputs=|++
  Out1 : Outport
  wires:
  e(t)/1 -> Gain1/1, S(t)/1(e(t))
  dX(t)/1 -> S(t)/2(dX(t))
  x(t)/1 -> Gain/1
  Gain/1 -> Sum/1
  Gain1/1 -> Sum/2
  S(t)/1(Out1) -> Divide/1, Abs/1
  Abs/1 -> Sum2/1
  Constant/1 -> Sum2/2
  Sum2/1 -> Divide/2
  Divide/1 -> Gain3/1
  Gain3/1 -> Sum1/1
  Sum1/1 -> Out1/1
  Sum/1 -> Gain2/1
  Gain2/1 -> Sum1/2

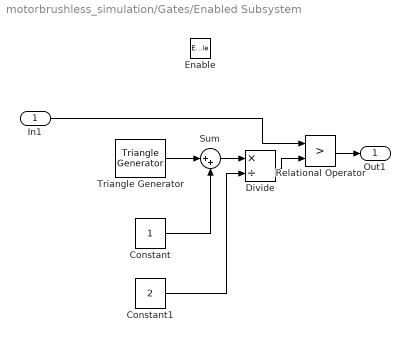
== system motorbrushless_simulation/Gates/Enabled Subsystem ==
  In1 : Inport
  Enable : EnablePort
  Constant : Constant
  Constant1 : Constant  Value=2
  Divide : Product  Inputs=*/
  Relational Operator : RelationalOperator  Operator=>  OutDataTypeStr=boolean
  Sum : Sum  Inputs=|++
  Triangle Generator : powerlib_meascontrol/Pulse & Signal Generators/Triangle Generator  Freq=4e3  Phase=90  Ts=Ts
  Out1 : Outport
  wires:
  Triangle Generator/1 -> Sum/1
  Constant/1 -> Sum/2
  Sum/1 -> Divide/1
  Divide/1 -> Relational Operator/2
  Constant1/1 -> Divide/2
  In1/1 -> Relational Operator/1
  Relational Operator/1 -> Out1/1

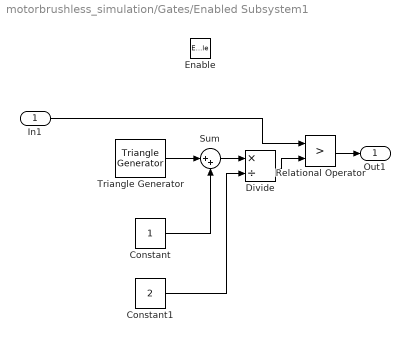
== system motorbrushless_simulation/Gates/Enabled Subsystem1 ==
  In1 : Inport
  Enable : EnablePort
  Constant : Constant
  Constant1 : Constant  Value=2
  Divide : Product  Inputs=*/
  Relational Operator : RelationalOperator  Operator=>  OutDataTypeStr=boolean
  Sum : Sum  Inputs=|++
  Triangle Generator : powerlib_meascontrol/Pulse & Signal Generators/Triangle Generator  Freq=4e3  Phase=90  Ts=Ts
  Out1 : Outport
  wires:
  Triangle Generator/1 -> Sum/1
  Constant/1 -> Sum/2
  Sum/1 -> Divide/1
  Divide/1 -> Relational Operator/2
  Constant1/1 -> Divide/2
  In1/1 -> Relational Operator/1
  Relational Operator/1 -> Out1/1

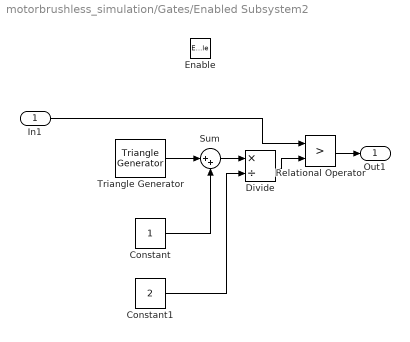
== system motorbrushless_simulation/Gates/Enabled Subsystem2 ==
  In1 : Inport
  Enable : EnablePort
  Constant : Constant
  Constant1 : Constant  Value=2
  Divide : Product  Inputs=*/
  Relational Operator : RelationalOperator  Operator=>  OutDataTypeStr=boolean
  Sum : Sum  Inputs=|++
  Triangle Generator : powerlib_meascontrol/Pulse & Signal Generators/Triangle Generator  Freq=4e3  Phase=90  Ts=Ts
  Out1 : Outport
  wires:
  Triangle Generator/1 -> Sum/1
  Constant/1 -> Sum/2
  Sum/1 -> Divide/1
  Divide/1 -> Relational Operator/2
  Constant1/1 -> Divide/2
  In1/1 -> Relational Operator/1
  Relational Operator/1 -> Out1/1

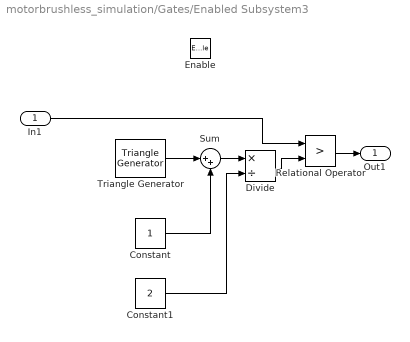
== system motorbrushless_simulation/Gates/Enabled Subsystem3 ==
  In1 : Inport
  Enable : EnablePort
  Constant : Constant
  Constant1 : Constant  Value=2
  Divide : Product  Inputs=*/
  Relational Operator : RelationalOperator  Operator=>  OutDataTypeStr=boolean
  Sum : Sum  Inputs=|++
  Triangle Generator : powerlib_meascontrol/Pulse & Signal Generators/Triangle Generator  Freq=4e3  Phase=90  Ts=Ts
  Out1 : Outport
  wires:
  Triangle Generator/1 -> Sum/1
  Constant/1 -> Sum/2
  Sum/1 -> Divide/1
  Divide/1 -> Relational Operator/2
  Constant1/1 -> Divide/2
  In1/1 -> Relational Operator/1
  Relational Operator/1 -> Out1/1

== system motorbrushless_simulation/Gates/Enabled Subsystem4 ==
  In1 : Inport
  Enable : EnablePort
  Constant : Constant
  Constant1 : Constant  Value=2
  Divide : Product  Inputs=*/
  Relational Operator : RelationalOperator  Operator=>  OutDataTypeStr=boolean
  Sum : Sum  Inputs=|++
  Triangle Generator : powerlib_meascontrol/Pulse & Signal Generators/Triangle Generator  Freq=4e3  Phase=90  Ts=Ts
  Out1 : Outport
  wires:
  Triangle Generator/1 -> Sum/1
  Constant/1 -> Sum/2
  Sum/1 -> Divide/1
  Divide/1 -> Relational Operator/2
  Constant1/1 -> Divide/2
  In1/1 -> Relational Operator/1
  Relational Operator/1 -> Out1/1

== system motorbrushless_simulation/Gates/Enabled Subsystem5 ==
  In1 : Inport
  Enable : EnablePort
  Constant : Constant
  Constant1 : Constant  Value=2
  Divide : Product  Inputs=*/
  Relational Operator : RelationalOperator  Operator=>  OutDataTypeStr=boolean
  Sum : Sum  Inputs=|++
  Triangle Generator : powerlib_meascontrol/Pulse & Signal Generators/Triangle Generator  Freq=4e3  Phase=90  Ts=Ts
  Out1 : Outport
  wires:
  Triangle Generator/1 -> Sum/1
  Constant/1 -> Sum/2
  Sum/1 -> Divide/1
  Divide/1 -> Relational Operator/2
  Constant1/1 -> Divide/2
  In1/1 -> Relational Operator/1
  Relational Operator/1 -> Out1/1

== system motorbrushless_simulation/Gates1/Enabled Subsystem ==
  In1 : Inport
  Enable : EnablePort
  Constant : Constant
  Constant1 : Constant  Value=2
  Divide : Product  Inputs=*/
  Relational Operator : RelationalOperator  Operator=>  OutDataTypeStr=boolean
  Sum : Sum  Inputs=|++
  Triangle Generator : powerlib_meascontrol/Pulse & Signal Generators/Triangle Generator  Freq=4e3  Phase=90  Ts=Ts
  Out1 : Outport
  wires:
  Triangle Generator/1 -> Sum/1
  Constant/1 -> Sum/2
  Sum/1 -> Divide/1
  Divide/1 -> Relational Operator/2
  Constant1/1 -> Divide/2
  In1/1 -> Relational Operator/1
  Relational Operator/1 -> Out1/1

== system motorbrushless_simulation/Gates1/Enabled Subsystem1 ==
  In1 : Inport
  Enable : EnablePort
  Constant : Constant
  Constant1 : Constant  Value=2
  Divide : Product  Inputs=*/
  Relational Operator : RelationalOperator  Operator=>  OutDataTypeStr=boolean
  Sum : Sum  Inputs=|++
  Triangle Generator : powerlib_meascontrol/Pulse & Signal Generators/Triangle Generator  Freq=4e3  Phase=90  Ts=Ts
  Out1 : Outport
  wires:
  Triangle Generator/1 -> Sum/1
  Constant/1 -> Sum/2
  Sum/1 -> Divide/1
  Divide/1 -> Relational Operator/2
  Constant1/1 -> Divide/2
  In1/1 -> Relational Operator/1
  Relational Operator/1 -> Out1/1

== system motorbrushless_simulation/Gates1/Enabled Subsystem2 ==
  In1 : Inport
  Enable : EnablePort
  Constant : Constant
  Constant1 : Constant  Value=2
  Divide : Product  Inputs=*/
  Relational Operator : RelationalOperator  Operator=>  OutDataTypeStr=boolean
  Sum : Sum  Inputs=|++
  Triangle Generator : powerlib_meascontrol/Pulse & Signal Generators/Triangle Generator  Freq=4e3  Phase=90  Ts=Ts
  Out1 : Outport
  wires:
  Triangle Generator/1 -> Sum/1
  Constant/1 -> Sum/2
  Sum/1 -> Divide/1
  Divide/1 -> Relational Operator/2
  Constant1/1 -> Divide/2
  In1/1 -> Relational Operator/1
  Relational Operator/1 -> Out1/1

== system motorbrushless_simulation/Gates1/Enabled Subsystem3 ==
  In1 : Inport
  Enable : EnablePort
  Constant : Constant
  Constant1 : Constant  Value=2
  Divide : Product  Inputs=*/
  Relational Operator : RelationalOperator  Operator=>  OutDataTypeStr=boolean
  Sum : Sum  Inputs=|++
  Triangle Generator : powerlib_meascontrol/Pulse & Signal Generators/Triangle Generator  Freq=4e3  Phase=90  Ts=Ts
  Out1 : Outport
  wires:
  Triangle Generator/1 -> Sum/1
  Constant/1 -> Sum/2
  Sum/1 -> Divide/1
  Divide/1 -> Relational Operator/2
  Constant1/1 -> Divide/2
  In1/1 -> Relational Operator/1
  Relational Operator/1 -> Out1/1

== system motorbrushless_simulation/Gates1/Enabled Subsystem4 ==
  In1 : Inport
  Enable : EnablePort
  Constant : Constant
  Constant1 : Constant  Value=2
  Divide : Product  Inputs=*/
  Relational Operator : RelationalOperator  Operator=>  OutDataTypeStr=boolean
  Sum : Sum  Inputs=|++
  Triangle Generator : powerlib_meascontrol/Pulse & Signal Generators/Triangle Generator  Freq=4e3  Phase=90  Ts=Ts
  Out1 : Outport
  wires:
  Triangle Generator/1 -> Sum/1
  Constant/1 -> Sum/2
  Sum/1 -> Divide/1
  Divide/1 -> Relational Operator/2
  Constant1/1 -> Divide/2
  In1/1 -> Relational Operator/1
  Relational Operator/1 -> Out1/1

== system motorbrushless_simulation/Gates1/Enabled Subsystem5 ==
  In1 : Inport
  Enable : EnablePort
  Constant : Constant
  Constant1 : Constant  Value=2
  Divide : Product  Inputs=*/
  Relational Operator : RelationalOperator  Operator=>  OutDataTypeStr=boolean
  Sum : Sum  Inputs=|++
  Triangle Generator : powerlib_meascontrol/Pulse & Signal Generators/Triangle Generator  Freq=4e3  Phase=90  Ts=Ts
  Out1 : Outport
  wires:
  Triangle Generator/1 -> Sum/1
  Constant/1 -> Sum/2
  Sum/1 -> Divide/1
  Divide/1 -> Relational Operator/2
  Constant1/1 -> Divide/2
  In1/1 -> Relational Operator/1
  Relational Operator/1 -> Out1/1

== system motorbrushless_simulation/Gates2/Enabled Subsystem ==
  In1 : Inport
  Enable : EnablePort
  Constant : Constant
  Constant1 : Constant  Value=2
  Divide : Product  Inputs=*/
  Relational Operator : RelationalOperator  Operator=>  OutDataTypeStr=boolean
  Sum : Sum  Inputs=|++
  Triangle Generator : powerlib_meascontrol/Pulse & Signal Generators/Triangle Generator  Freq=4e3  Phase=90  Ts=Ts
  Out1 : Outport
  wires:
  Triangle Generator/1 -> Sum/1
  Constant/1 -> Sum/2
  Sum/1 -> Divide/1
  Divide/1 -> Relational Operator/2
  Constant1/1 -> Divide/2
  In1/1 -> Relational Operator/1
  Relational Operator/1 -> Out1/1

== system motorbrushless_simulation/Gates2/Enabled Subsystem1 ==
  In1 : Inport
  Enable : EnablePort
  Constant : Constant
  Constant1 : Constant  Value=2
  Divide : Product  Inputs=*/
  Relational Operator : RelationalOperator  Operator=>  OutDataTypeStr=boolean
  Sum : Sum  Inputs=|++
  Triangle Generator : powerlib_meascontrol/Pulse & Signal Generators/Triangle Generator  Freq=4e3  Phase=90  Ts=Ts
  Out1 : Outport
  wires:
  Triangle Generator/1 -> Sum/1
  Constant/1 -> Sum/2
  Sum/1 -> Divide/1
  Divide/1 -> Relational Operator/2
  Constant1/1 -> Divide/2
  In1/1 -> Relational Operator/1
  Relational Operator/1 -> Out1/1

== system motorbrushless_simulation/Gates2/Enabled Subsystem2 ==
  In1 : Inport
  Enable : EnablePort
  Constant : Constant
  Constant1 : Constant  Value=2
  Divide : Product  Inputs=*/
  Relational Operator : RelationalOperator  Operator=>  OutDataTypeStr=boolean
  Sum : Sum  Inputs=|++
  Triangle Generator : powerlib_meascontrol/Pulse & Signal Generators/Triangle Generator  Freq=4e3  Phase=90  Ts=Ts
  Out1 : Outport
  wires:
  Triangle Generator/1 -> Sum/1
  Constant/1 -> Sum/2
  Sum/1 -> Divide/1
  Divide/1 -> Relational Operator/2
  Constant1/1 -> Divide/2
  In1/1 -> Relational Operator/1
  Relational Operator/1 -> Out1/1

== system motorbrushless_simulation/Gates2/Enabled Subsystem3 ==
  In1 : Inport
  Enable : EnablePort
  Constant : Constant
  Constant1 : Constant  Value=2
  Divide : Product  Inputs=*/
  Relational Operator : RelationalOperator  Operator=>  OutDataTypeStr=boolean
  Sum : Sum  Inputs=|++
  Triangle Generator : powerlib_meascontrol/Pulse & Signal Generators/Triangle Generator  Freq=4e3  Phase=90  Ts=Ts
  Out1 : Outport
  wires:
  Triangle Generator/1 -> Sum/1
  Constant/1 -> Sum/2
  Sum/1 -> Divide/1
  Divide/1 -> Relational Operator/2
  Constant1/1 -> Divide/2
  In1/1 -> Relational Operator/1
  Relational Operator/1 -> Out1/1

== system motorbrushless_simulation/Gates2/Enabled Subsystem4 ==
  In1 : Inport
  Enable : EnablePort
  Constant : Constant
  Constant1 : Constant  Value=2
  Divide : Product  Inputs=*/
  Relational Operator : RelationalOperator  Operator=>  OutDataTypeStr=boolean
  Sum : Sum  Inputs=|++
  Triangle Generator : powerlib_meascontrol/Pulse & Signal Generators/Triangle Generator  Freq=4e3  Phase=90  Ts=Ts
  Out1 : Outport
  wires:
  Triangle Generator/1 -> Sum/1
  Constant/1 -> Sum/2
  Sum/1 -> Divide/1
  Divide/1 -> Relational Operator/2
  Constant1/1 -> Divide/2
  In1/1 -> Relational Operator/1
  Relational Operator/1 -> Out1/1

== system motorbrushless_simulation/Gates2/Enabled Subsystem5 ==
  In1 : Inport
  Enable : EnablePort
  Constant : Constant
  Constant1 : Constant  Value=2
  Divide : Product  Inputs=*/
  Relational Operator : RelationalOperator  Operator=>  OutDataTypeStr=boolean
  Sum : Sum  Inputs=|++
  Triangle Generator : powerlib_meascontrol/Pulse & Signal Generators/Triangle Generator  Freq=4e3  Phase=90  Ts=Ts
  Out1 : Outport
  wires:
  Triangle Generator/1 -> Sum/1
  Constant/1 -> Sum/2
  Sum/1 -> Divide/1
  Divide/1 -> Relational Operator/2
  Constant1/1 -> Divide/2
  In1/1 -> Relational Operator/1
  Relational Operator/1 -> Out1/1

== system motorbrushless_simulation/SMC1/S(t) ==
  e(t) : Inport
  dX(t) : Inport  Port=2
  Gain : Gain  Gain=3256.96
  Gain1 : Gain  Gain=12e6
  Gain2 : Gain  Gain=-1
  Integrator : Integrator
  Sum : Sum  Inputs=|+++
  Out1 : Outport
  wires:
  Gain/1 -> Sum/1
  e(t)/1 -> Integrator/1, Gain/1
  Gain1/1 -> Sum/2
  Integrator/1 -> Gain1/1
  Sum/1 -> Out1/1
  dX(t)/1 -> Gain2/1
  Gain2/1 -> Sum/3
